simulink model "CleanerGroup3"  (R2024b)
settings: Solver=VariableStepAuto  StartTime=0.0  StopTime=inf  RelTol=1e-3
undefined symbols (not defined in the file): boxes, circles, dock, dockWidth, tMax
libraries: sfRobotExampleLib x4
(part 2 of 2)

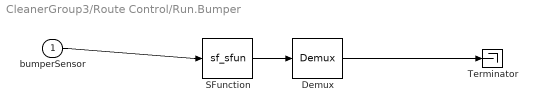
== system CleanerGroup3/Route Control/Run.Bumper ==
  bumperSensor : Inport
  " Demux " : Demux  Outputs=1
  " SFunction " : S-Function  Tag=Stateflow S-Function 2  FunctionName=sf_sfun  PortCounts=[1 1]  SFunctionDeploymentMode=off  EnableBusSupport=on
  " Terminator " : Terminator
  wires:
  bumperSensor/1 -> " SFunction "/1
  " Demux "/1 -> " Terminator "/1
  " SFunction "/1 -> " Demux "/1

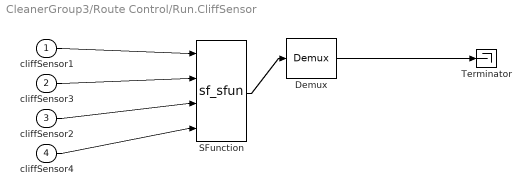
== system CleanerGroup3/Route Control/Run.CliffSensor ==
  cliffSensor1 : Inport
  cliffSensor3 : Inport  Port=2
  cliffSensor2 : Inport  Port=3
  cliffSensor4 : Inport  Port=4
  " Demux " : Demux  Outputs=1
  " SFunction " : S-Function  Tag=Stateflow S-Function 5  FunctionName=sf_sfun  PortCounts=[4 1]  SFunctionDeploymentMode=off  EnableBusSupport=on
  " Terminator " : Terminator
  wires:
  cliffSensor1/1 -> " SFunction "/1
  cliffSensor3/1 -> " SFunction "/2
  cliffSensor2/1 -> " SFunction "/3
  cliffSensor4/1 -> " SFunction "/4
  " Demux "/1 -> " Terminator "/1
  " SFunction "/1 -> " Demux "/1

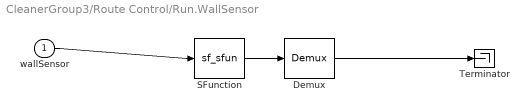
== system CleanerGroup3/Route Control/Run.WallSensor ==
  wallSensor : Inport
  " Demux " : Demux  Outputs=1
  " SFunction " : S-Function  Tag=Stateflow S-Function 4  FunctionName=sf_sfun  PortCounts=[1 1]  SFunctionDeploymentMode=off  EnableBusSupport=on
  " Terminator " : Terminator
  wires:
  wallSensor/1 -> " SFunction "/1
  " Demux "/1 -> " Terminator "/1
  " SFunction "/1 -> " Demux "/1

== stateflow chart CleanerGroup3/Route Control/Run.Bumper ==
  state Bumber
    if bumperSensor==1
    direction = -1;
    else
    direction = 1;
    end
    Robot.rotate(direction*45)
  (default) -> Bumber
  Bumber -> 29
  data: direction local; bumperSensor input

== stateflow chart CleanerGroup3/Route Control ==
  state Run
    state Bumper
    state CliffSensor
    state WallSensor
    state Move
    state ContactDock
    state Rotate
    Move -> Bumper [order 2] : [bumperSensor > 0 ]
    151 -> Move
    (junction 201) -> WallSensor
    (junction 203) -> CliffSensor
    161 -> (junction 192)
    184 -> (junction 198)
    180 -> (junction 205)
    (default) -> Move : {speed = 0.5;}
    Move -> (junction 203) [order 3] : [cliffSensor1 == 1 || cliffSensor2 == 1 || cliffSensor3 == 1 || cliffSensor4 == 1]
    Move -> (junction 201) [order 1] : [wallSensor < 10]
    108 -> (junction 120)
    (junction 121) -> Move
    (junction 122) -> (junction 121)
    (junction 120) -> (junction 124)
    (junction 123) -> (junction 121) [order 2]
    (junction 119) -> (junction 122) : {speed = 0.1;}
    107 -> ContactDock
    112 -> (junction 123)
    (junction 123) -> (junction 119) [order 1] : [distToDock < 2]
    (junction 125) -> (junction 123)
    111 -> (junction 207)
    (junction 205) -> (junction 207)
    (junction 207) -> 116
    (junction 198) -> (junction 124)
    (junction 124) -> 115
    117 -> (junction 125)
    (junction 195) -> (junction 124)
    (junction 192) -> (junction 195)
  state Stop
    done = true;
  (default) -> Run
  Run -> Stop [order 1] : [distToDock<dockWidth]
  Run -> Stop [order 2] : after(tMax,sec)
      | {coder.extrinsic('warning');
      | warning('Unable to reach dock.');}
  data: speed function_input; distToDock function_output; distToDock local double size=1 =Inf; speed local double size=1; tMax parameter; done output boolean size=1 =false; dockWidth parameter; bumperSensor input; wallSensor input; cliffSensor1 input; cliffSensor2 input; cliffSensor3 input; cliffSensor4 input

== stateflow chart CleanerGroup3/Route Control/Run.WallSensor ==
  state Wall
    if wallSensor>10
    direction = 1;
    else
    direction = -1;
    end
    Robot.move(direction*0.5);
  (default) -> Wall
  Wall -> 2
  data: direction local; wallSensor input

== stateflow chart CleanerGroup3/Route Control/Run.CliffSensor ==
  state Cliff
    if cliffSensor1 == 1 || cliffSensor2 == 1
    direction = -1;
    next = 1;
    elseif cliffSensor3 == 1 || cliffSensor4 == 1
    direction = -1;
    next = 2;
    else
    direction = 0;
    next = 0;
    end
    Robot.move(direction * 0.5);
  state LeftSideSensor
  state RightSideSensor
  (default) -> Cliff
  Cliff -> LeftSideSensor [order 1] : [next >= 2]
  Cliff -> RightSideSensor [order 2]
  LeftSideSensor -> 18
  RightSideSensor -> 20
  data: cliffSensor1 input; cliffSensor3 input; cliffSensor2 input; cliffSensor4 input; direction local; next local

== stateflow chart CleanerGroup3/Plot Trajectory1 ==
  state Init
    coder.extrinsic('sfRobotScene','plot','hold');
    sfRobotScene(dock,dockWidth,boxes,circles);
    xPrev = x;
    yPrev = y;
  state Plot
    plot([xPrev,x],[yPrev,y],'ob');
    xPrev = x;
    yPrev = y;
  state End
    plot([xPrev,x],[yPrev,y],'ob');
    stop = true;
  (default) -> Init
  Init -> Plot
  Plot -> End : [done]
  data: dock parameter double size=[1 2]; boxes parameter; circles parameter; xPrev local double size=1; yPrev local double size=1; x input; y input; done input boolean size=1; stop output boolean =false; dockWidth parameter double size=1
